simulink model "Ejemplo_3_Dead_Reckoning2"  (R2022a)
settings: Solver=FixedStepDiscrete  StartTime=0.0  StopTime=10  FixedStep=0.01  RelTol=1e-3
undefined symbols (not defined in the file or in its folder): ticksPerRot, wheelR
libraries: mobileRoboticsTrainingLib x3
settings Model: Creator=L03107259  LastModifiedBy=L03107259

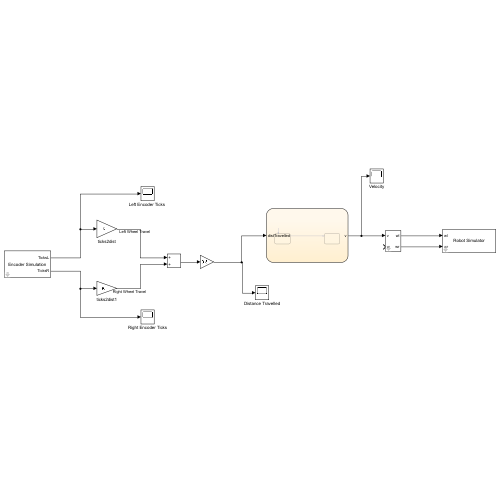
[thumbnail: Simulink's stored preview of the top-level diagram]
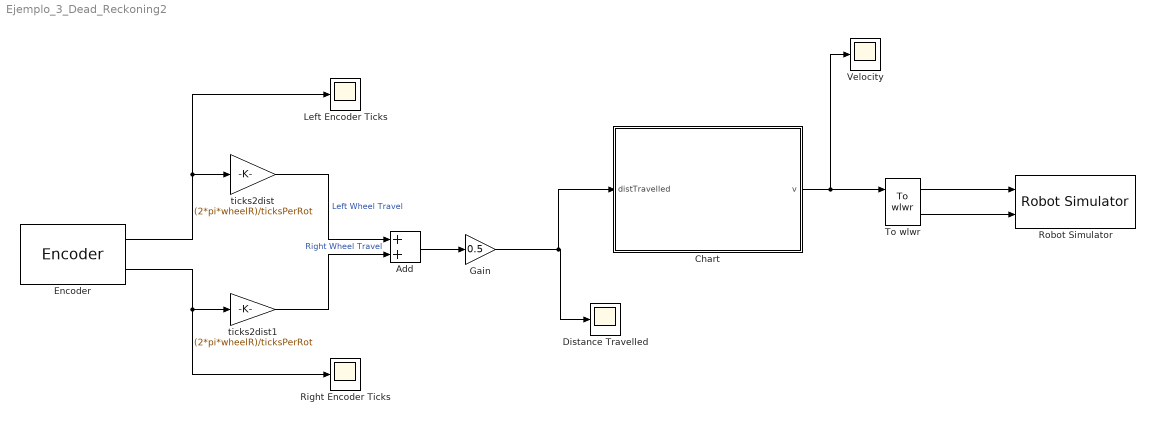
== system Ejemplo_3_Dead_Reckoning2 ==
  Add : Sum
  Chart : Stateflow chart  TreatAsAtomicUnit=on
  Distance Travelled : Scope
  Encoder : mobileRoboticsTrainingLib/Encoder  axleLength=axleLength  wheelR=wheelR  ticksPerRot=ticksPerRot
      settings: SourceProductName=Mobile Robotics Training Library
  Gain : Gain  Gain=0.5
  "Left Encoder Ticks " : Scope
  Right Encoder Ticks : Scope
  Robot Simulator : mobileRoboticsTrainingLib/Robot Simulator  Priority=99  mapVar=[]  startX=1  startY=1  startTheta=0  axleLength=axleLength  wheelR=wheelR
  To wlwr : mobileRoboticsTrainingLib/To wlwr  axleLength=axleLength  wheelR=wheelR
  Velocity : Scope
  ticks2dist : Gain  Gain=(2*pi*wheelR)/ticksPerRot
  ticks2dist1 : Gain  Gain=(2*pi*wheelR)/ticksPerRot
  wires:
  Encoder/1 -> "Left Encoder Ticks "/1, ticks2dist/1
  ticks2dist/1 -> Add/1  "Left Wheel Travel"
  ticks2dist1/1 -> Add/2  "Right Wheel Travel"
  Encoder/2 -> Right Encoder Ticks/1, ticks2dist1/1
  Add/1 -> Gain/1
  Gain/1 -> Chart/1(distTravelled), Distance Travelled/1
  Chart/1(v) -> To wlwr/1, Velocity/1
  To wlwr/1 -> Robot Simulator/1
  To wlwr/2 -> Robot Simulator/2

== stateflow chart Ejemplo_3_Dead_Reckoning2/Chart ==
  state MoveForward
    entry: v=0.1;
  state Stop
    entry: v=0;
  (default) -> MoveForward : % Start
  MoveForward -> Stop : [distTravelled>=1]
  data: distTravelled input; v output
